simulink model "Eleven_Blocked_Rotor_Test_on_IM"  (R2024a)
settings: Solver=VariableStepAuto  StartTime=0.0  StopTime=5  RelTol=1e-3
libraries: spsACVoltageSourceLib x3, spsCurrentMeasurementLib x3, spsVoltageMeasurementLib x3, spsRMSLib x2, spsAsynchronousMachineSIUnitsLib x1, spsPowerLib x1, sps_lib x1
settings Model: Creator=91889  LastModifiedBy=91889
settings DataIOCC: InitialState=[0 0 0 0 0 0 0 0 0 0 0 0 0 0 0 0 0 0 0 0 0 0 0 0 0]  LoadInitialState=on

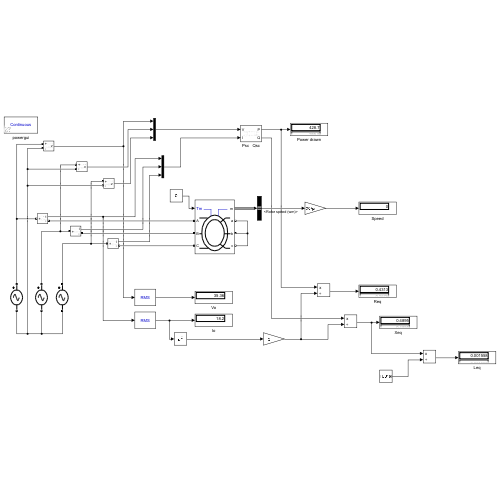
[thumbnail: Simulink's stored preview of the top-level diagram]
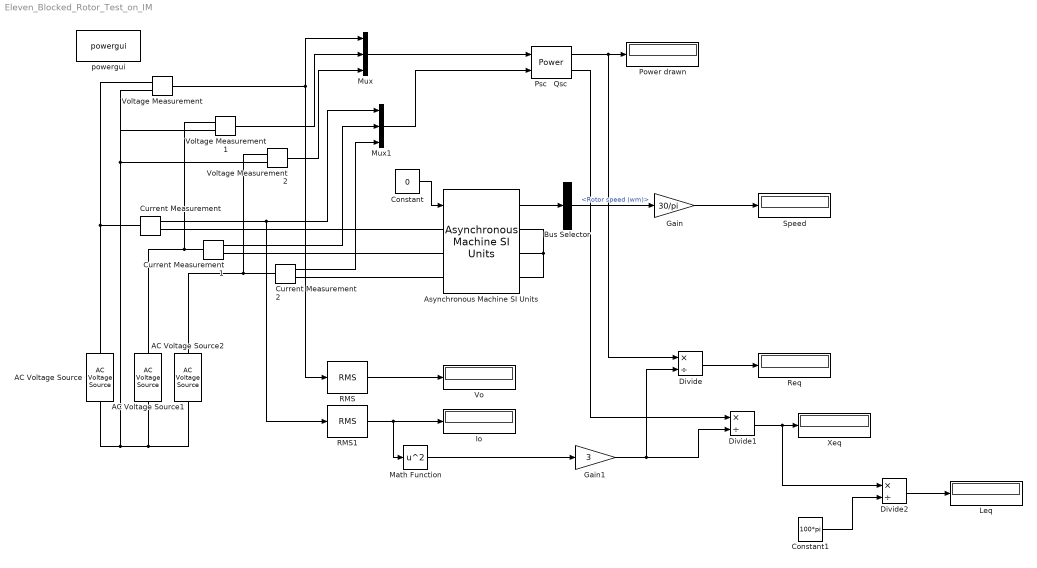
== system Eleven_Blocked_Rotor_Test_on_IM ==
  AC Voltage Source : spsACVoltageSourceLib/AC Voltage Source  Amplitude=50  Phase=0  Frequency=50  SampleTime=0  Measurements=None  BusType=swing  Pref=10e3  Qref=0  Qmin=-inf  Qmax=+inf
  AC Voltage Source1 : spsACVoltageSourceLib/AC Voltage Source  Amplitude=50  Phase=-120  Frequency=50  SampleTime=0  Measurements=None  BusType=swing  Pref=10e3  Qref=0  Qmin=-inf  Qmax=+inf
  AC Voltage Source2 : spsACVoltageSourceLib/AC Voltage Source  Amplitude=50  Phase=120  Frequency=50  SampleTime=0  Measurements=None  BusType=swing  Pref=10e3  Qref=0  Qmin=-inf  Qmax=+inf
  Asynchronous Machine SI Units : spsAsynchronousMachineSIUnitsLib/Asynchronous Machine SI Units  RotorType=Wound  PresetModel=No  MechanicalLoad=Torque Tm  ShowDetailedParameters=on  ReferenceFrame=Rotor  Units=SI  MeasurementBus=off  NominalParameters=[1.845e+04 400 50]  VoltageRatio=1  Stator=[0.5968 0.0003495]  Rotor=[0.6258 0.005473]  Cage1=[0.4155 0.002066]  Cage2=[0.4168 0.0003495]  Lm=0.0354  Mechanical=[inf 0.005879 2]  PolePairs=2  InitialConditions=[0 0 0 0 0 0 0 0]  SimulateSaturation=off  Saturation=[14.03593122, 27.81365428, 53.79336849, 72.68890987, 97.98006896, 148.6815601, 215.7428561, 302.9841135, 428.7778367 ; 230, 322, 414, 460, 506, 552, 598, 644, 690]  LoadFlowParameters=1492000  TsPowergui=0  TsBlock=-1  IterativeModel=Trapezoidal non iterative  IterativeDiscreteModel=Trapezoidal non iterative  Pmec=1.492e+006
  Bus Selector : BusSelector  OutputSignals=Mechanical.Rotor speed (wm)
  Constant : Constant  Value=0
  Constant1 : Constant  Value=100*pi
  Current Measurement : spsCurrentMeasurementLib/Current Measurement  PhasorSimulation=off  OutputType=Complex  PSBequivalent=0
  Current Measurement1 : spsCurrentMeasurementLib/Current Measurement  PhasorSimulation=off  OutputType=Complex  PSBequivalent=0
  Current Measurement2 : spsCurrentMeasurementLib/Current Measurement  PhasorSimulation=off  OutputType=Complex  PSBequivalent=0
  Divide : Product  Inputs=*/
  Divide1 : Product  Inputs=*/
  Divide2 : Product  Inputs=*/
  Gain : Gain  Gain=30/pi
  Gain1 : Gain  Gain=3
  Io : Display
  Leq : Display
  Math Function : Math  Operator=square
  Mux : Mux  Inputs=3
  Mux1 : Mux  Inputs=3
  Power drawn : Display
  Psc   Qsc : spsPowerLib/Power  Freq=60  Vinit=[1, 0]  Iinit=[1, 0]  Ts=0
  RMS : spsRMSLib/RMS  TrueRMS=on  Freq=50  RMSInit=0  Ts=0
  RMS1 : spsRMSLib/RMS  TrueRMS=on  Freq=50  RMSInit=0  Ts=0
  Req : Display
  Speed : Display
  Vo : Display
  Voltage Measurement : spsVoltageMeasurementLib/Voltage Measurement  PhasorSimulation=off  OutputType=Complex  PSBequivalent=0
  Voltage Measurement1 : spsVoltageMeasurementLib/Voltage Measurement  PhasorSimulation=off  OutputType=Complex  PSBequivalent=0
  Voltage Measurement2 : spsVoltageMeasurementLib/Voltage Measurement  PhasorSimulation=off  OutputType=Complex  PSBequivalent=0
  Xeq : Display
  powergui : sps_lib/powergui  Priority=1  SimulationMode=Continuous  SampleTime=50e-6  frequency=60  Iterations=50  frequencyindice=50  Pbase=100e6  ErrMax=1e-4  UnitsV=kV  UnitsW=MW  buscounter=0  FunctionMessages=off  echomessages=off  EnableUseOfTLC=off  CurrentSourceSwitches=off  DisableSnubberDevices=off  DisableRonSwitches=off  DisableVfSwitches=off  DisplayEquations=off  AutomaticDiscreteSolvers=off  SolverType=Tustin/Backward Euler (TBE)  Interpol=off  ExternalGateDelay=off  methode=off  Ts=100  x0status=blocks  SPID=on  SwTol=0  HookPort=off  NonlinearTolerance=1e-4  nMaxIteration=100  ContinueOnMaxIteration=off  RestoreLinks=warning  ResistiveCurrentMeasurement=off  Frange=[0:2:500]  Ylog=off  Xlog=on  ShowGrid=off  save=off  variable=ZData  structure=0  ZoomFFT=off  StartTime=0.0  cycles=1  DisplayStyle=1  fundamental=60  FreqAxis=off  MaxFrequency=1000  frequencyindicesteady=1  RmsSteady=1  display=off
  wires:
  Current Measurement/1 -> RMS1/1, Mux1/1
  RMS1/1 -> Math Function/1, Io/1
  Voltage Measurement1/1 -> Mux/2
  Voltage Measurement/1 -> RMS/1, Mux/1
  Current Measurement1/1 -> Mux1/2
  Mux1/1 -> Psc   Qsc/2
  Bus Selector/1 -> Gain/1  "<Rotor speed (wm)>"
  Asynchronous Machine SI Units/1 -> Bus Selector/1
  Voltage Measurement2/1 -> Mux/3
  Constant/1 -> Asynchronous Machine SI Units/1
  Psc   Qsc/1 -> Divide/1, Power drawn/1
  Gain/1 -> Speed/1
  RMS/1 -> Vo/1
  Mux/1 -> Psc   Qsc/1
  Current Measurement2/1 -> Mux1/3
  Math Function/1 -> Gain1/1
  Divide/1 -> Req/1
  Gain1/1 -> Divide1/2, Divide/2
  Psc   Qsc/2 -> Divide1/1
  Divide1/1 -> Divide2/1, Xeq/1
  Constant1/1 -> Divide2/2
  Divide2/1 -> Leq/1
  connections:
  AC Voltage Source/LConn1 -- Voltage Measurement2/LConn2 -- Voltage Measurement1/LConn2 -- Voltage Measurement/LConn2 -- AC Voltage Source1/LConn1 -- AC Voltage Source2/LConn1
  Asynchronous Machine SI Units/RConn1 -- Asynchronous Machine SI Units/RConn2 -- Asynchronous Machine SI Units/RConn3
  Current Measurement2/LConn1 -- AC Voltage Source2/RConn1 -- Voltage Measurement2/LConn1
  Current Measurement/LConn1 -- AC Voltage Source/RConn1 -- Voltage Measurement/LConn1
  Current Measurement1/LConn1 -- AC Voltage Source1/RConn1 -- Voltage Measurement1/LConn1
  Current Measurement2/RConn1 -- Asynchronous Machine SI Units/LConn3
  Current Measurement1/RConn1 -- Asynchronous Machine SI Units/LConn2
  Current Measurement/RConn1 -- Asynchronous Machine SI Units/LConn1
